simulink model "simuexo4"  (R2020b)
settings: Solver=VariableStepAuto  StartTime=0.0  StopTime=0.5  MaxStep=0.0001  RelTol=1e-3
undefined symbols (not defined in the file or in its folder): Fs, Rs
libraries: simulink x3
settings Model: Creator=Etudiants  LastModifiedBy=Etudiants

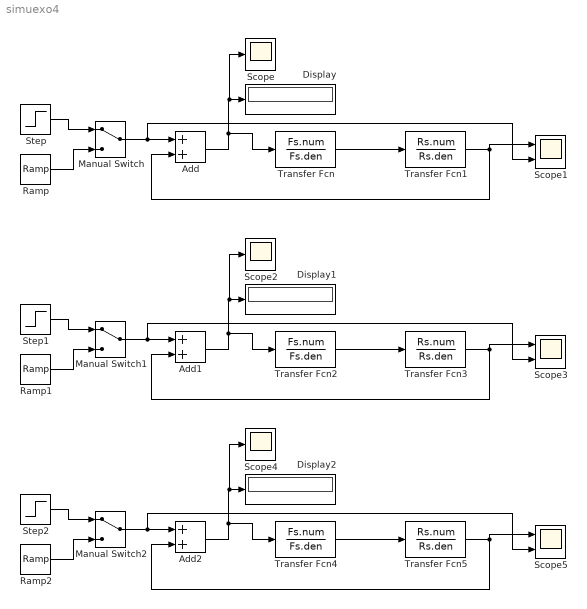
== system simuexo4 ==
  Add : Sum
  Add1 : Sum
  Add2 : Sum
  Display : Display
  Display1 : Display
  Display2 : Display
  Manual Switch : ManualSwitch
  Manual Switch1 : ManualSwitch
  Manual Switch2 : ManualSwitch
  Ramp : simulink/Sources/Ramp  slope=1  start=0  InitialOutput=0
  Ramp1 : simulink/Sources/Ramp  slope=1  start=0  InitialOutput=0
  Ramp2 : simulink/Sources/Ramp  slope=1  start=0  InitialOutput=0
  Scope : Scope
  Scope1 : Scope  NumInputPorts=2
  Scope2 : Scope
  Scope3 : Scope  NumInputPorts=2
  Scope4 : Scope
  Scope5 : Scope  NumInputPorts=2
  Step : Step  Time=0  After=10  SampleTime=0
  Step1 : Step  Time=0  After=10  SampleTime=0
  Step2 : Step  Time=0  After=10  SampleTime=0
  Transfer Fcn : TransferFcn  Numerator=Fs.num  Denominator=Fs.den
  Transfer Fcn1 : TransferFcn  Numerator=Rs.num  Denominator=Rs.den
  Transfer Fcn2 : TransferFcn  Numerator=Fs.num  Denominator=Fs.den
  Transfer Fcn3 : TransferFcn  Numerator=Rs.num  Denominator=Rs.den
  Transfer Fcn4 : TransferFcn  Numerator=Fs.num  Denominator=Fs.den
  Transfer Fcn5 : TransferFcn  Numerator=Rs.num  Denominator=Rs.den
  wires:
  Step/1 -> Manual Switch/1
  Ramp/1 -> Manual Switch/2
  Manual Switch/1 -> Add/1, Scope1/2
  Add/1 -> Transfer Fcn/1, Scope/1, Display/1
  Transfer Fcn/1 -> Transfer Fcn1/1
  Transfer Fcn1/1 -> Add/2, Scope1/1
  Transfer Fcn2/1 -> Transfer Fcn3/1
  Transfer Fcn3/1 -> Add1/2, Scope3/1
  Manual Switch1/1 -> Add1/1, Scope3/2
  Ramp1/1 -> Manual Switch1/2
  Step1/1 -> Manual Switch1/1
  Add1/1 -> Transfer Fcn2/1, Scope2/1, Display1/1
  Transfer Fcn4/1 -> Transfer Fcn5/1
  Transfer Fcn5/1 -> Add2/2, Scope5/1
  Manual Switch2/1 -> Add2/1, Scope5/2
  Ramp2/1 -> Manual Switch2/2
  Step2/1 -> Manual Switch2/1
  Add2/1 -> Transfer Fcn4/1, Scope4/1, Display2/1
